simulink model "test5"  (Simulink 8.4)
settings: Solver=ode45  StartTime=0.0  StopTime=10.0  RelTol=1e-3
libraries: simulink x1
settings Model: Creator=GM  LastModifiedBy=GM
settings DataIOCC: LimitDataPoints=off  SignalLoggingSaveFormat=Dataset
settings OptimizationCC: ExpressionDepthLimit=128  LifeSpan=auto
settings DebuggingCC: UnderspecifiedInitializationDetection=Simplified  MergeDetectMultiDrivingBlocksExec=error  SolverPrmCheckMsg=none  FcnCallInpInsideContextMsg=EnableAllAsWarning  FrameProcessingCompatibilityMsg=error  StateNameClashWarn=none  SFUnexpectedBacktrackingDiag=error  SFNoUnconditionalDefaultTransitionDiag=error
settings HardwareCC: ProdBitPerPointer=64  ProdLargestAtomicFloat=Float  ProdIntDivRoundTo=Zero  ProdEndianess=LittleEndian  ProdWordSize=64  ProdHWDeviceType=Intel->x86-64 (Windows64)
settings ModelReferenceCC: PropagateSignalLabelsOutOfModel=on
settings GRTTargetCC: GeneratePreprocessorConditionals=Use local settings  CombineOutputUpdateFcns=on  GRTInterface=off

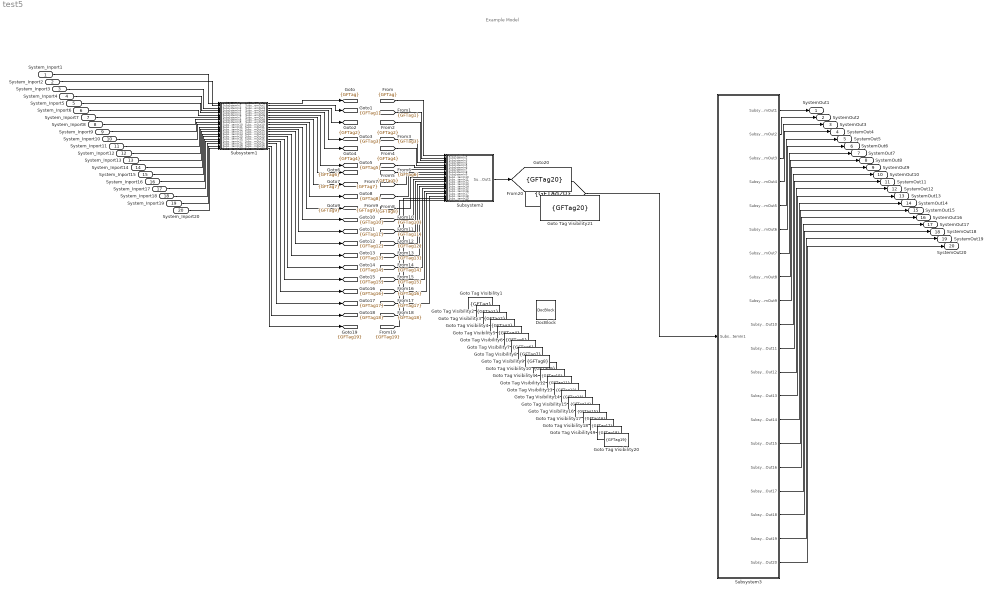
== system test5 ==
  note: Example Model
  System_Inport1 : Inport  OutDataTypeStr=single
  System_Inport2 : Inport  Port=2  OutDataTypeStr=single
  System_Inport3 : Inport  Port=3  OutDataTypeStr=single
  System_Inport4 : Inport  Port=4  OutDataTypeStr=single
  System_Inport5 : Inport  Port=5  OutDataTypeStr=single
  System_Inport6 : Inport  Port=6  OutDataTypeStr=single
  System_Inport7 : Inport  Port=7  OutDataTypeStr=single
  System_Inport8 : Inport  Port=8  OutDataTypeStr=single
  System_Inport9 : Inport  Port=9  OutDataTypeStr=single
  System_Inport10 : Inport  Port=10  OutDataTypeStr=single
  System_Inport11 : Inport  Port=11  OutDataTypeStr=single
  System_Inport12 : Inport  Port=12  OutDataTypeStr=single
  System_Inport13 : Inport  Port=13  OutDataTypeStr=single
  System_Inport14 : Inport  Port=14  OutDataTypeStr=single
  System_Inport15 : Inport  Port=15  OutDataTypeStr=single
  System_Inport16 : Inport  Port=16  OutDataTypeStr=single
  System_Inport17 : Inport  Port=17  OutDataTypeStr=single
  System_Inport18 : Inport  Port=18  OutDataTypeStr=single
  System_Inport19 : Inport  Port=19  OutDataTypeStr=single
  System_Inport20 : Inport  Port=20  OutDataTypeStr=single
  DocBlock : simulink/Model-Wide Utilities/DocBlock  ECoderFlag=DocBlock  DocumentType=RTF
  Goto Tag Visibility1 : GotoTagVisibility  GotoTag=GFTag
  Goto Tag Visibility10 : GotoTagVisibility  GotoTag=GFTag9
  Goto Tag Visibility11 : GotoTagVisibility  GotoTag=GFTag10
  Goto Tag Visibility12 : GotoTagVisibility  GotoTag=GFTag11
  Goto Tag Visibility13 : GotoTagVisibility  GotoTag=GFTag12
  Goto Tag Visibility14 : GotoTagVisibility  GotoTag=GFTag13
  Goto Tag Visibility15 : GotoTagVisibility  GotoTag=GFTag14
  Goto Tag Visibility16 : GotoTagVisibility  GotoTag=GFTag15
  Goto Tag Visibility17 : GotoTagVisibility  GotoTag=GFTag16
  Goto Tag Visibility18 : GotoTagVisibility  GotoTag=GFTag17
  Goto Tag Visibility19 : GotoTagVisibility  GotoTag=GFTag18
  Goto Tag Visibility2 : GotoTagVisibility  GotoTag=GFTag1
  Goto Tag Visibility20 : GotoTagVisibility  GotoTag=GFTag19
  Goto Tag Visibility21 : GotoTagVisibility  GotoTag=GFTag20
  Goto Tag Visibility3 : GotoTagVisibility  GotoTag=GFTag2
  Goto Tag Visibility4 : GotoTagVisibility  GotoTag=GFTag3
  Goto Tag Visibility5 : GotoTagVisibility  GotoTag=GFTag4
  Goto Tag Visibility6 : GotoTagVisibility  GotoTag=GFTag5
  Goto Tag Visibility7 : GotoTagVisibility  GotoTag=GFTag6
  Goto Tag Visibility8 : GotoTagVisibility  GotoTag=GFTag7
  Goto Tag Visibility9 : GotoTagVisibility  GotoTag=GFTag8
  Subsystem1 : Subsystem  AncestorBlock=ESSR/ESSR/ESSI
  Subsystem2 : Subsystem  AncestorBlock=ESSR/ESSR/ESSI
  Subsystem3 : Subsystem  AncestorBlock=ESSR/ESSR/Controller Output
  SystemOut1 : Outport
  SystemOut2 : Outport  Port=2
  SystemOut3 : Outport  Port=3
  SystemOut4 : Outport  Port=4
  SystemOut5 : Outport  Port=5
  SystemOut6 : Outport  Port=6
  SystemOut7 : Outport  Port=7
  SystemOut8 : Outport  Port=8
  SystemOut9 : Outport  Port=9
  SystemOut10 : Outport  Port=10
  SystemOut11 : Outport  Port=11
  SystemOut12 : Outport  Port=12
  SystemOut13 : Outport  Port=13
  SystemOut14 : Outport  Port=14
  SystemOut15 : Outport  Port=15
  SystemOut16 : Outport  Port=16
  SystemOut17 : Outport  Port=17
  SystemOut18 : Outport  Port=18
  SystemOut19 : Outport  Port=19
  SystemOut20 : Outport  Port=20
  tag scope: GFTag10=scoped, GFTag11=scoped, GFTag12=scoped, GFTag13=scoped, GFTag14=scoped, GFTag15=scoped, GFTag16=scoped, GFTag17=scoped, GFTag18=scoped, GFTag19=scoped, GFTag1=scoped, GFTag20=scoped, GFTag2=scoped, GFTag3=scoped, GFTag4=scoped, GFTag5=scoped, GFTag6=scoped, GFTag7=scoped, GFTag8=scoped, GFTag9=scoped, GFTag=scoped
  wires:
  Subsystem2/1(SubsystemOut1) -> [GFTag20]
  Subsystem3/1(SubsystemOut1) -> SystemOut1/1
  Subsystem3/2(SubsystemOut2) -> SystemOut2/1
  Subsystem3/3(SubsystemOut3) -> SystemOut3/1
  Subsystem3/4(SubsystemOut4) -> SystemOut4/1
  Subsystem3/5(SubsystemOut5) -> SystemOut5/1
  Subsystem3/6(SubsystemOut6) -> SystemOut6/1
  Subsystem3/7(SubsystemOut7) -> SystemOut7/1
  Subsystem3/8(SubsystemOut8) -> SystemOut8/1
  Subsystem3/9(SubsystemOut9) -> SystemOut9/1
  Subsystem3/10(SubsystemOut10) -> SystemOut10/1
  Subsystem3/11(SubsystemOut11) -> SystemOut11/1
  Subsystem3/12(SubsystemOut12) -> SystemOut12/1
  Subsystem3/13(SubsystemOut13) -> SystemOut13/1
  Subsystem3/14(SubsystemOut14) -> SystemOut14/1
  Subsystem3/15(SubsystemOut15) -> SystemOut15/1
  Subsystem3/16(SubsystemOut16) -> SystemOut16/1
  Subsystem3/17(SubsystemOut17) -> SystemOut17/1
  Subsystem3/18(SubsystemOut18) -> SystemOut18/1
  Subsystem3/19(SubsystemOut19) -> SystemOut19/1
  Subsystem3/20(SubsystemOut20) -> SystemOut20/1
  [GFTag20] -> Subsystem3/1(SubsystemIn1)
  [GFTag5] -> Subsystem2/6(SubsystemIn6)
  [GFTag6] -> Subsystem2/7(SubsystemIn7)
  [GFTag7] -> Subsystem2/8(SubsystemIn8)
  [GFTag4] -> Subsystem2/5(SubsystemIn5)
  [GFTag8] -> Subsystem2/9(SubsystemIn9)
  [GFTag3] -> Subsystem2/4(SubsystemIn4)
  [GFTag9] -> Subsystem2/10(SubsystemIn10)
  [GFTag2] -> Subsystem2/3(SubsystemIn3)
  [GFTag10] -> Subsystem2/11(SubsystemIn11)
  [GFTag1] -> Subsystem2/2(SubsystemIn2)
  [GFTag11] -> Subsystem2/12(SubsystemIn12)
  [GFTag] -> Subsystem2/1(SubsystemIn1)
  [GFTag12] -> Subsystem2/13(SubsystemIn13)
  [GFTag13] -> Subsystem2/14(SubsystemIn14)
  [GFTag14] -> Subsystem2/15(SubsystemIn15)
  [GFTag15] -> Subsystem2/16(SubsystemIn16)
  [GFTag16] -> Subsystem2/17(SubsystemIn17)
  [GFTag17] -> Subsystem2/18(SubsystemIn18)
  [GFTag18] -> Subsystem2/19(SubsystemIn19)
  [GFTag19] -> Subsystem2/20(SubsystemIn20)
  System_Inport20/1 -> Subsystem1/20(SubsystemIn20)
  System_Inport19/1 -> Subsystem1/19(SubsystemIn19)
  System_Inport18/1 -> Subsystem1/18(SubsystemIn18)
  System_Inport17/1 -> Subsystem1/17(SubsystemIn17)
  System_Inport16/1 -> Subsystem1/16(SubsystemIn16)
  System_Inport15/1 -> Subsystem1/15(SubsystemIn15)
  System_Inport14/1 -> Subsystem1/14(SubsystemIn14)
  System_Inport13/1 -> Subsystem1/13(SubsystemIn13)
  System_Inport12/1 -> Subsystem1/12(SubsystemIn12)
  System_Inport11/1 -> Subsystem1/11(SubsystemIn11)
  System_Inport10/1 -> Subsystem1/10(SubsystemIn10)
  System_Inport9/1 -> Subsystem1/9(SubsystemIn9)
  System_Inport8/1 -> Subsystem1/8(SubsystemIn8)
  System_Inport7/1 -> Subsystem1/7(SubsystemIn7)
  System_Inport6/1 -> Subsystem1/6(SubsystemIn6)
  System_Inport5/1 -> Subsystem1/5(SubsystemIn5)
  System_Inport4/1 -> Subsystem1/4(SubsystemIn4)
  System_Inport3/1 -> Subsystem1/3(SubsystemIn3)
  System_Inport2/1 -> Subsystem1/2(SubsystemIn2)
  System_Inport1/1 -> Subsystem1/1(SubsystemIn1)
  Subsystem1/1(SubsystemOut1) -> [GFTag]
  Subsystem1/2(SubsystemOut2) -> [GFTag1]
  Subsystem1/3(SubsystemOut3) -> [GFTag2]
  Subsystem1/4(SubsystemOut4) -> [GFTag3]
  Subsystem1/5(SubsystemOut5) -> [GFTag4]
  Subsystem1/6(SubsystemOut6) -> [GFTag5]
  Subsystem1/7(SubsystemOut7) -> [GFTag6]
  Subsystem1/8(SubsystemOut8) -> [GFTag7]
  Subsystem1/9(SubsystemOut9) -> [GFTag8]
  Subsystem1/10(SubsystemOut10) -> [GFTag9]
  Subsystem1/11(SubsystemOut11) -> [GFTag10]
  Subsystem1/12(SubsystemOut12) -> [GFTag11]
  Subsystem1/13(SubsystemOut13) -> [GFTag12]
  Subsystem1/14(SubsystemOut14) -> [GFTag13]
  Subsystem1/15(SubsystemOut15) -> [GFTag14]
  Subsystem1/16(SubsystemOut16) -> [GFTag15]
  Subsystem1/17(SubsystemOut17) -> [GFTag16]
  Subsystem1/18(SubsystemOut18) -> [GFTag17]
  Subsystem1/19(SubsystemOut19) -> [GFTag18]
  Subsystem1/20(SubsystemOut20) -> [GFTag19]

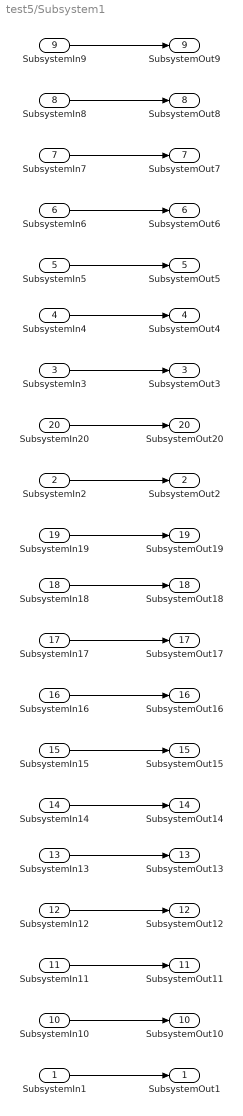
== system test5/Subsystem1 ==
  SubsystemIn1 : Inport
  SubsystemIn2 : Inport  Port=2
  SubsystemIn3 : Inport  Port=3
  SubsystemIn4 : Inport  Port=4
  SubsystemIn5 : Inport  Port=5
  SubsystemIn6 : Inport  Port=6
  SubsystemIn7 : Inport  Port=7
  SubsystemIn8 : Inport  Port=8
  SubsystemIn9 : Inport  Port=9
  SubsystemIn10 : Inport  Port=10
  SubsystemIn11 : Inport  Port=11
  SubsystemIn12 : Inport  Port=12
  SubsystemIn13 : Inport  Port=13
  SubsystemIn14 : Inport  Port=14
  SubsystemIn15 : Inport  Port=15
  SubsystemIn16 : Inport  Port=16
  SubsystemIn17 : Inport  Port=17
  SubsystemIn18 : Inport  Port=18
  SubsystemIn19 : Inport  Port=19
  SubsystemIn20 : Inport  Port=20
  SubsystemOut1 : Outport
  SubsystemOut2 : Outport  Port=2
  SubsystemOut3 : Outport  Port=3
  SubsystemOut4 : Outport  Port=4
  SubsystemOut5 : Outport  Port=5
  SubsystemOut6 : Outport  Port=6
  SubsystemOut7 : Outport  Port=7
  SubsystemOut8 : Outport  Port=8
  SubsystemOut9 : Outport  Port=9
  SubsystemOut10 : Outport  Port=10
  SubsystemOut11 : Outport  Port=11
  SubsystemOut12 : Outport  Port=12
  SubsystemOut13 : Outport  Port=13
  SubsystemOut14 : Outport  Port=14
  SubsystemOut15 : Outport  Port=15
  SubsystemOut16 : Outport  Port=16
  SubsystemOut17 : Outport  Port=17
  SubsystemOut18 : Outport  Port=18
  SubsystemOut19 : Outport  Port=19
  SubsystemOut20 : Outport  Port=20
  wires:
  SubsystemIn1/1 -> SubsystemOut1/1
  SubsystemIn2/1 -> SubsystemOut2/1
  SubsystemIn3/1 -> SubsystemOut3/1
  SubsystemIn4/1 -> SubsystemOut4/1
  SubsystemIn5/1 -> SubsystemOut5/1
  SubsystemIn6/1 -> SubsystemOut6/1
  SubsystemIn7/1 -> SubsystemOut7/1
  SubsystemIn8/1 -> SubsystemOut8/1
  SubsystemIn9/1 -> SubsystemOut9/1
  SubsystemIn10/1 -> SubsystemOut10/1
  SubsystemIn11/1 -> SubsystemOut11/1
  SubsystemIn12/1 -> SubsystemOut12/1
  SubsystemIn13/1 -> SubsystemOut13/1
  SubsystemIn14/1 -> SubsystemOut14/1
  SubsystemIn15/1 -> SubsystemOut15/1
  SubsystemIn16/1 -> SubsystemOut16/1
  SubsystemIn17/1 -> SubsystemOut17/1
  SubsystemIn18/1 -> SubsystemOut18/1
  SubsystemIn19/1 -> SubsystemOut19/1
  SubsystemIn20/1 -> SubsystemOut20/1

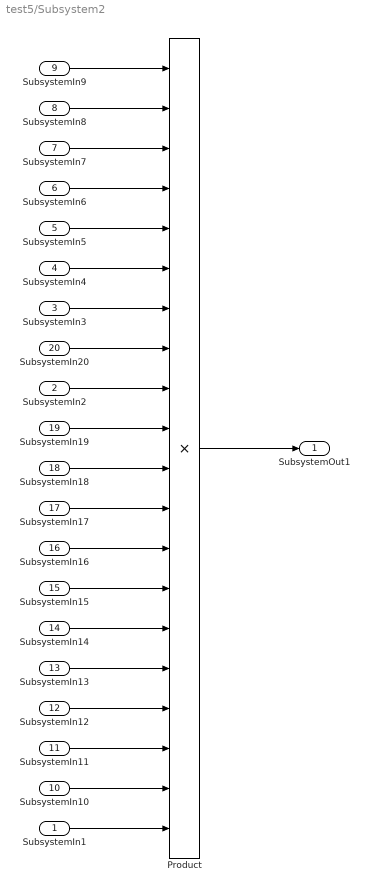
== system test5/Subsystem2 ==
  SubsystemIn1 : Inport
  SubsystemIn2 : Inport  Port=2
  SubsystemIn3 : Inport  Port=3
  SubsystemIn4 : Inport  Port=4
  SubsystemIn5 : Inport  Port=5
  SubsystemIn6 : Inport  Port=6
  SubsystemIn7 : Inport  Port=7
  SubsystemIn8 : Inport  Port=8
  SubsystemIn9 : Inport  Port=9
  SubsystemIn10 : Inport  Port=10
  SubsystemIn11 : Inport  Port=11
  SubsystemIn12 : Inport  Port=12
  SubsystemIn13 : Inport  Port=13
  SubsystemIn14 : Inport  Port=14
  SubsystemIn15 : Inport  Port=15
  SubsystemIn16 : Inport  Port=16
  SubsystemIn17 : Inport  Port=17
  SubsystemIn18 : Inport  Port=18
  SubsystemIn19 : Inport  Port=19
  SubsystemIn20 : Inport  Port=20
  Product : Product  Inputs=20
  SubsystemOut1 : Outport
  wires:
  SubsystemIn9/1 -> Product/1
  SubsystemIn8/1 -> Product/2
  SubsystemIn7/1 -> Product/3
  SubsystemIn6/1 -> Product/4
  SubsystemIn5/1 -> Product/5
  SubsystemIn4/1 -> Product/6
  SubsystemIn3/1 -> Product/7
  SubsystemIn20/1 -> Product/8
  SubsystemIn2/1 -> Product/9
  SubsystemIn19/1 -> Product/10
  SubsystemIn18/1 -> Product/11
  SubsystemIn17/1 -> Product/12
  SubsystemIn16/1 -> Product/13
  SubsystemIn15/1 -> Product/14
  SubsystemIn14/1 -> Product/15
  SubsystemIn13/1 -> Product/16
  SubsystemIn12/1 -> Product/17
  SubsystemIn11/1 -> Product/18
  SubsystemIn10/1 -> Product/19
  SubsystemIn1/1 -> Product/20
  Product/1 -> SubsystemOut1/1

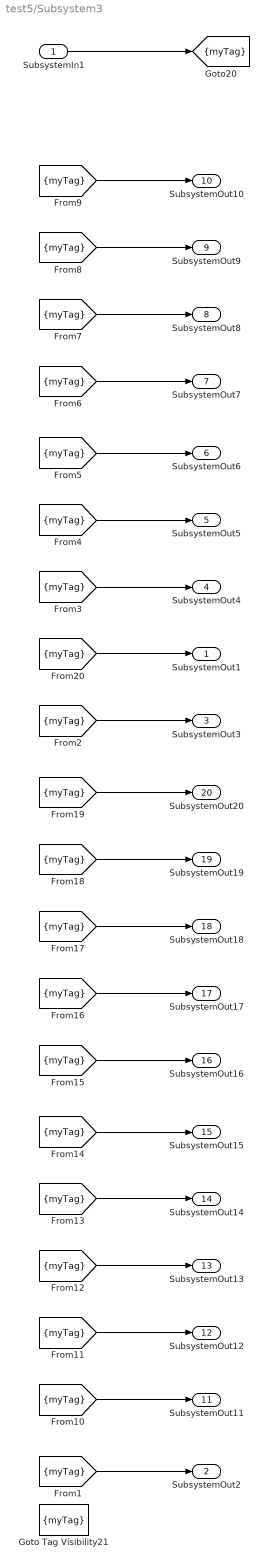
== system test5/Subsystem3 ==
  SubsystemIn1 : Inport
  Goto Tag Visibility21 : GotoTagVisibility  GotoTag=myTag
  SubsystemOut1 : Outport
  SubsystemOut2 : Outport  Port=2
  SubsystemOut3 : Outport  Port=3
  SubsystemOut4 : Outport  Port=4
  SubsystemOut5 : Outport  Port=5
  SubsystemOut6 : Outport  Port=6
  SubsystemOut7 : Outport  Port=7
  SubsystemOut8 : Outport  Port=8
  SubsystemOut9 : Outport  Port=9
  SubsystemOut10 : Outport  Port=10
  SubsystemOut11 : Outport  Port=11
  SubsystemOut12 : Outport  Port=12
  SubsystemOut13 : Outport  Port=13
  SubsystemOut14 : Outport  Port=14
  SubsystemOut15 : Outport  Port=15
  SubsystemOut16 : Outport  Port=16
  SubsystemOut17 : Outport  Port=17
  SubsystemOut18 : Outport  Port=18
  SubsystemOut19 : Outport  Port=19
  SubsystemOut20 : Outport  Port=20
  tag scope: myTag=scoped
  wires:
  SubsystemIn1/1 -> [myTag]
  [myTag] -> SubsystemOut1/1
  [myTag] -> SubsystemOut2/1
  [myTag] -> SubsystemOut3/1
  [myTag] -> SubsystemOut4/1
  [myTag] -> SubsystemOut5/1
  [myTag] -> SubsystemOut6/1
  [myTag] -> SubsystemOut7/1
  [myTag] -> SubsystemOut8/1
  [myTag] -> SubsystemOut9/1
  [myTag] -> SubsystemOut10/1
  [myTag] -> SubsystemOut11/1
  [myTag] -> SubsystemOut12/1
  [myTag] -> SubsystemOut13/1
  [myTag] -> SubsystemOut14/1
  [myTag] -> SubsystemOut15/1
  [myTag] -> SubsystemOut16/1
  [myTag] -> SubsystemOut17/1
  [myTag] -> SubsystemOut18/1
  [myTag] -> SubsystemOut19/1
  [myTag] -> SubsystemOut20/1
